simulink model "travel_control_2017"  (R2017b)
settings: Solver=VariableStepAuto  StartTime=0.0  StopTime=20  RelTol=1e-3
values from neighbouring files (symbols this model uses):
  ddotLambda_P_den = J_t    (= 1.06056619635)    [controller_params.m]
  ddotLambda_P_num = L_a * F_steady    (= 2.3872825)    [controller_params.m]
  ddotP_deltaF_den = J_p    (= 0.044886917226)    [controller_params.m]
  ddotP_deltaF_num = L_h    (= 0.177419)    [controller_params.m]
  deltaF_max = 3    [controller_params.m]
libraries: simulink x4
settings Model: Creator=bryankikuta  LastModifiedBy=bryankikuta
settings DataIOCC: ReturnWorkspaceOutputs=on
settings DebuggingCC: UnconnectedInputMsg=none  UnconnectedOutputMsg=none  UnconnectedLineMsg=none
settings ModelReferenceCC: EnableRefExpFcnMdlSchedulingChecks=off
settings SFSimCC: SimUseLocalCustomCode=on
settings RTWCC: Description=Generic Real-Time Target  RTWUseLocalCustomCode=on

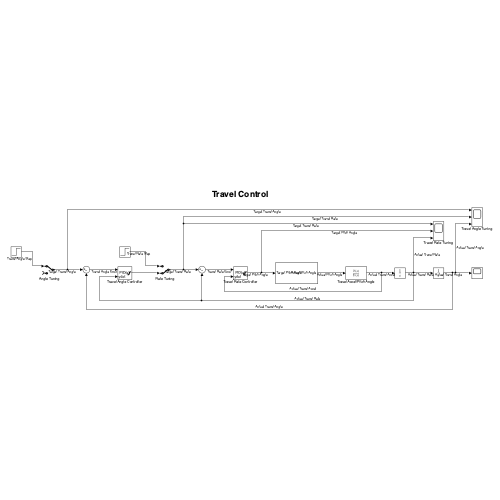
[thumbnail: Simulink's stored preview of the top-level diagram]
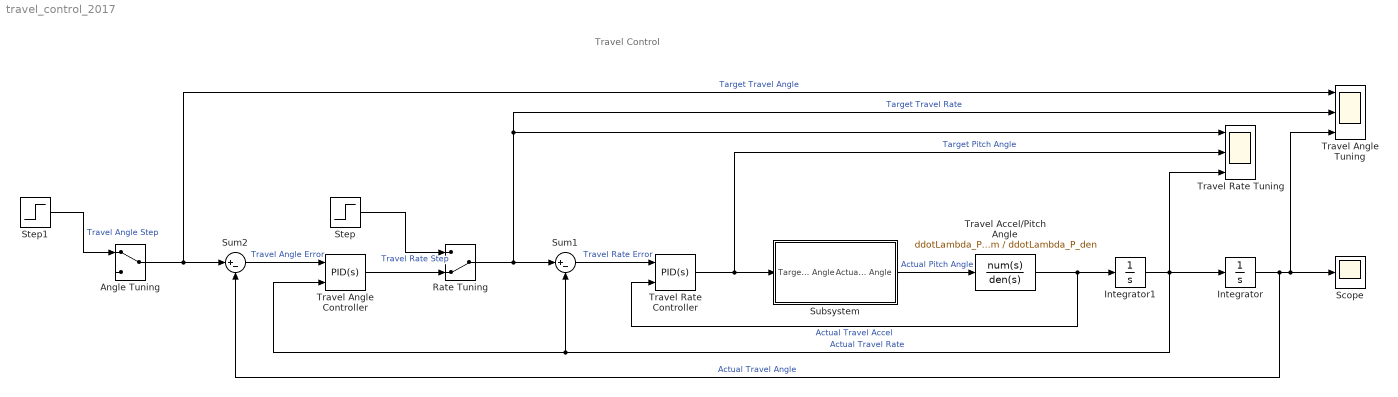
== system travel_control_2017 ==
  note: Travel Control
  Angle Tuning : ManualSwitch
  Integrator : Integrator
  Integrator1 : Integrator
  Rate Tuning : ManualSwitch  CurrentSetting=0
  Scope : Scope
  Step : Step  After=45 * pi/180  SampleTime=0
  Step1 : Step  After=pi  SampleTime=0
  Subsystem : Subsystem
  Sum1 : Sum  Inputs=|+-
  Sum2 : Sum  Inputs=|+-
  Travel Accel/Pitch Angle : TransferFcn  Numerator=ddotLambda_P_num  Denominator=ddotLambda_P_den
  Travel Angle Controller : simulink/Continuous/PID Controller  Controller=PID  Form=Parallel  TimeDomain=Continuous-time  SampleTime=-1  IntegratorMethod=Forward Euler  FilterMethod=Forward Euler  ControllerParametersSource=internal  P=0.5  I=0  D=.4  N=3.1657121688489  UseFilter=on  TunerSelectOption=Transfer Function Based (PID Tuner App)  InitialConditionSource=internal  InitialConditionForIntegrator=0  InitialConditionForFilter=0  DifferentiatorICPrevScaledInput=0  ExternalReset=none  TrackingMode=off  Kt=1  LimitOutput=on  UpperSaturationLimit=45 * pi/180  LowerSaturationLimit=-45 * pi/180  LinearizeAsGain=off  AntiWindupMode=none  Kb=1  POutMin=[]  POutMax=[]  IOutMin=[]  IOutMax=[]  DOutMin=[]  DOutMax=[]  NOutMin=[]  NOutMax=[]  SumOutMin=[]  SumOutMax=[]  SaturationOutMin=[]  SaturationOutMax=[]  PParamMin=[]  PParamMax=[]  IParamMin=[]  IParamMax=[]  DParamMin=[]  DParamMax=[]  NParamMin=[]  NParamMax=[]  KbParamMin=[]  KbParamMax=[]  KtParamMin=[]  KtParamMax=[]  KbOutMin=[]  KbOutMax=[]  KtOutMin=[]  KtOutMax=[]  IntegratorOutMin=[]  IntegratorOutMax=[]  FilterOutMin=[]  FilterOutMax=[]  SumI1OutMin=[]  SumI1OutMax=[]  SumI2OutMin=[]  SumI2OutMax=[]  SumI3OutMin=[]  SumI3OutMax=[]  SumDOutMin=[]  SumDOutMax=[]  DifferentiatorOutMin=[]  DifferentiatorOutMax=[]  FilterDiffOutCoefMin=[]  FilterDiffOutCoefMax=[]  ReciprocalOutMin=[]  ReciprocalOutMax=[]  SumDenOutMin=[]  SumDenOutMax=[]  SumNumOutMin=[]  SumNumOutMax=[]  DivideOutMin=[]  DivideOutMax=[]  IntegratorContinuousStateAttributes=''  IntegratorStateMustResolveToSignalObject=off  IntegratorRTWStateStorageClass=Auto  FilterContinuousStateAttributes=''  FilterStateMustResolveToSignalObject=off  FilterRTWStateStorageClass=Auto  InitialConditionSetting=State (most efficient)
  Travel Angle Tuning : Scope  NumInputPorts=3
  Travel Rate Controller : simulink/Continuous/PID Controller  Controller=PID  Form=Parallel  TimeDomain=Continuous-time  SampleTime=-1  IntegratorMethod=Forward Euler  FilterMethod=Forward Euler  ControllerParametersSource=internal  P=0.3  I=0.002  D=0.05  N=3.1657121688489  UseFilter=on  TunerSelectOption=Transfer Function Based (PID Tuner App)  InitialConditionSource=internal  InitialConditionForIntegrator=0  InitialConditionForFilter=0  DifferentiatorICPrevScaledInput=0  ExternalReset=none  TrackingMode=off  Kt=1  LimitOutput=on  UpperSaturationLimit=15 * pi/180  LowerSaturationLimit=-15 * pi/180  LinearizeAsGain=off  AntiWindupMode=none  Kb=1  POutMin=[]  POutMax=[]  IOutMin=[]  IOutMax=[]  DOutMin=[]  DOutMax=[]  NOutMin=[]  NOutMax=[]  SumOutMin=[]  SumOutMax=[]  SaturationOutMin=[]  SaturationOutMax=[]  PParamMin=[]  PParamMax=[]  IParamMin=[]  IParamMax=[]  DParamMin=[]  DParamMax=[]  NParamMin=[]  NParamMax=[]  KbParamMin=[]  KbParamMax=[]  KtParamMin=[]  KtParamMax=[]  KbOutMin=[]  KbOutMax=[]  KtOutMin=[]  KtOutMax=[]  IntegratorOutMin=[]  IntegratorOutMax=[]  FilterOutMin=[]  FilterOutMax=[]  SumI1OutMin=[]  SumI1OutMax=[]  SumI2OutMin=[]  SumI2OutMax=[]  SumI3OutMin=[]  SumI3OutMax=[]  SumDOutMin=[]  SumDOutMax=[]  DifferentiatorOutMin=[]  DifferentiatorOutMax=[]  FilterDiffOutCoefMin=[]  FilterDiffOutCoefMax=[]  ReciprocalOutMin=[]  ReciprocalOutMax=[]  SumDenOutMin=[]  SumDenOutMax=[]  SumNumOutMin=[]  SumNumOutMax=[]  DivideOutMin=[]  DivideOutMax=[]  IntegratorContinuousStateAttributes=''  IntegratorStateMustResolveToSignalObject=off  IntegratorRTWStateStorageClass=Auto  FilterContinuousStateAttributes=''  FilterStateMustResolveToSignalObject=off  FilterRTWStateStorageClass=Auto  InitialConditionSetting=State (most efficient)
  Travel Rate Tuning : Scope  NumInputPorts=3
  wires:
  Travel Rate Controller/1 -> Travel Rate Tuning/2, Subsystem/1(Target Pitch Angle)  "Target Pitch Angle"
  Sum1/1 -> Travel Rate Controller/1  "Travel Rate Error"
  Rate Tuning/1 -> Travel Rate Tuning/1, Travel Angle Tuning/2, Sum1/1  "Target Travel Rate"
  Subsystem/1(Actual Pitch Angle) -> Travel Accel/Pitch Angle/1  "Actual Pitch Angle"
  Travel Accel/Pitch Angle/1 -> Travel Rate Controller/2, Integrator1/1  "Actual Travel Accel"
  Travel Angle Controller/1 -> Rate Tuning/2
  Integrator/1 -> Travel Angle Tuning/3, Scope/1, Sum2/2  "Actual Travel Angle"
  Sum2/1 -> Travel Angle Controller/1  "Travel Angle Error"
  Angle Tuning/1 -> Sum2/1, Travel Angle Tuning/1  "Target Travel Angle"
  Step/1 -> Rate Tuning/1  "Travel Rate Step"
  Step1/1 -> Angle Tuning/1  "Travel Angle Step"
  Integrator1/1 -> Travel Rate Tuning/3, Integrator/1, Travel Angle Controller/2, Sum1/2  "Actual Travel Rate"

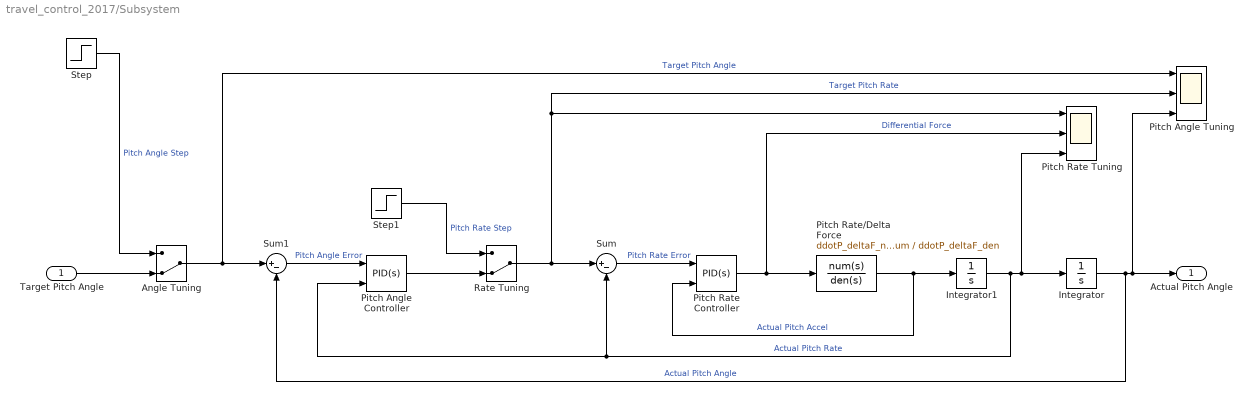
== system travel_control_2017/Subsystem ==
  Target Pitch Angle : Inport
  Angle Tuning : ManualSwitch  CurrentSetting=0
  Integrator : Integrator
  Integrator1 : Integrator
  Pitch Angle Controller : simulink/Continuous/PID Controller  Controller=PID  Form=Parallel  TimeDomain=Continuous-time  SampleTime=-1  IntegratorMethod=Forward Euler  FilterMethod=Forward Euler  ControllerParametersSource=internal  P=3  I=0  D=0.15  N=3.1657121688489  UseFilter=on  TunerSelectOption=Transfer Function Based (PID Tuner App)  InitialConditionSource=internal  InitialConditionForIntegrator=0  InitialConditionForFilter=0  DifferentiatorICPrevScaledInput=0  ExternalReset=none  TrackingMode=off  Kt=1  LimitOutput=on  UpperSaturationLimit=pi/2  LowerSaturationLimit=-pi/2  LinearizeAsGain=off  AntiWindupMode=none  Kb=1  POutMin=[]  POutMax=[]  IOutMin=[]  IOutMax=[]  DOutMin=[]  DOutMax=[]  NOutMin=[]  NOutMax=[]  SumOutMin=[]  SumOutMax=[]  SaturationOutMin=[]  SaturationOutMax=[]  PParamMin=[]  PParamMax=[]  IParamMin=[]  IParamMax=[]  DParamMin=[]  DParamMax=[]  NParamMin=[]  NParamMax=[]  KbParamMin=[]  KbParamMax=[]  KtParamMin=[]  KtParamMax=[]  KbOutMin=[]  KbOutMax=[]  KtOutMin=[]  KtOutMax=[]  IntegratorOutMin=[]  IntegratorOutMax=[]  FilterOutMin=[]  FilterOutMax=[]  SumI1OutMin=[]  SumI1OutMax=[]  SumI2OutMin=[]  SumI2OutMax=[]  SumI3OutMin=[]  SumI3OutMax=[]  SumDOutMin=[]  SumDOutMax=[]  DifferentiatorOutMin=[]  DifferentiatorOutMax=[]  FilterDiffOutCoefMin=[]  FilterDiffOutCoefMax=[]  ReciprocalOutMin=[]  ReciprocalOutMax=[]  SumDenOutMin=[]  SumDenOutMax=[]  SumNumOutMin=[]  SumNumOutMax=[]  DivideOutMin=[]  DivideOutMax=[]  IntegratorContinuousStateAttributes=''  IntegratorStateMustResolveToSignalObject=off  IntegratorRTWStateStorageClass=Auto  FilterContinuousStateAttributes=''  FilterStateMustResolveToSignalObject=off  FilterRTWStateStorageClass=Auto  InitialConditionSetting=State (most efficient)
  Pitch Angle Tuning : Scope  NumInputPorts=3
  Pitch Rate Controller : simulink/Continuous/PID Controller  Controller=PID  Form=Parallel  TimeDomain=Continuous-time  SampleTime=-1  IntegratorMethod=Forward Euler  FilterMethod=Forward Euler  ControllerParametersSource=internal  P=2  I=0.2  D=0.1  N=11.5322702769143  UseFilter=on  TunerSelectOption=Transfer Function Based (PID Tuner App)  InitialConditionSource=internal  InitialConditionForIntegrator=0  InitialConditionForFilter=0  DifferentiatorICPrevScaledInput=0  ExternalReset=none  TrackingMode=off  Kt=1  LimitOutput=on  UpperSaturationLimit=deltaF_max  LowerSaturationLimit=-deltaF_max  LinearizeAsGain=off  AntiWindupMode=none  Kb=1  POutMin=[]  POutMax=[]  IOutMin=[]  IOutMax=[]  DOutMin=[]  DOutMax=[]  NOutMin=[]  NOutMax=[]  SumOutMin=[]  SumOutMax=[]  SaturationOutMin=[]  SaturationOutMax=[]  PParamMin=[]  PParamMax=[]  IParamMin=[]  IParamMax=[]  DParamMin=[]  DParamMax=[]  NParamMin=[]  NParamMax=[]  KbParamMin=[]  KbParamMax=[]  KtParamMin=[]  KtParamMax=[]  KbOutMin=[]  KbOutMax=[]  KtOutMin=[]  KtOutMax=[]  IntegratorOutMin=[]  IntegratorOutMax=[]  FilterOutMin=[]  FilterOutMax=[]  SumI1OutMin=[]  SumI1OutMax=[]  SumI2OutMin=[]  SumI2OutMax=[]  SumI3OutMin=[]  SumI3OutMax=[]  SumDOutMin=[]  SumDOutMax=[]  DifferentiatorOutMin=[]  DifferentiatorOutMax=[]  FilterDiffOutCoefMin=[]  FilterDiffOutCoefMax=[]  ReciprocalOutMin=[]  ReciprocalOutMax=[]  SumDenOutMin=[]  SumDenOutMax=[]  SumNumOutMin=[]  SumNumOutMax=[]  DivideOutMin=[]  DivideOutMax=[]  IntegratorContinuousStateAttributes=''  IntegratorStateMustResolveToSignalObject=off  IntegratorRTWStateStorageClass=Auto  FilterContinuousStateAttributes=''  FilterStateMustResolveToSignalObject=off  FilterRTWStateStorageClass=Auto  InitialConditionSetting=State (most efficient)
  Pitch Rate Tuning : Scope  NumInputPorts=3
  Pitch Rate/Delta Force : TransferFcn  Numerator=ddotP_deltaF_num  Denominator=ddotP_deltaF_den
  Rate Tuning : ManualSwitch  CurrentSetting=0
  Step : Step  After=30 * pi/180  SampleTime=0
  Step1 : Step  Time=0  After=pi / 2  SampleTime=0
  Sum : Sum  Inputs=|+-
  Sum1 : Sum  Inputs=|+-
  Actual Pitch Angle : Outport
  wires:
  Target Pitch Angle/1 -> Angle Tuning/2
  Angle Tuning/1 -> Pitch Angle Tuning/1, Sum1/1  "Target Pitch Angle"
  Sum1/1 -> Pitch Angle Controller/1  "Pitch Angle Error"
  Step1/1 -> Rate Tuning/1  "Pitch Rate Step"
  Integrator/1 -> Actual Pitch Angle/1, Pitch Angle Tuning/3, Sum1/2  "Actual Pitch Angle"
  Rate Tuning/1 -> Pitch Angle Tuning/2, Pitch Rate Tuning/1, Sum/1  "Target Pitch Rate"
  Sum/1 -> Pitch Rate Controller/1  "Pitch Rate Error"
  Pitch Rate Controller/1 -> Pitch Rate Tuning/2, Pitch Rate/Delta Force/1  "Differential Force"
  Step/1 -> Angle Tuning/1  "Pitch Angle Step"
  Pitch Angle Controller/1 -> Rate Tuning/2
  Pitch Rate/Delta Force/1 -> Pitch Rate Controller/2, Integrator1/1  "Actual Pitch Accel"
  Integrator1/1 -> Pitch Rate Tuning/3, Integrator/1, Pitch Angle Controller/2, Sum/2  "Actual Pitch Rate"
